simulink library "carnot"  (R2013b)
settings: Solver=ode45  StartTime=0.0  StopTime=10.0  RelTol=1e-3
undefined symbols (not defined in the file or in its folder): A, acol, Ahabit, Awin, Azimuth_Angle, AziWin, B, C, c1, c4, capc, caph, CarnotCallbacks_Density, CarnotCallbacks_Enthalpy, CarnotCallbacks_Enthalpy2Temperature, CarnotCallbacks_Entropy, CarnotCallbacks_Evaporation_Enthalpy, CarnotCallbacks_GlobalMessageLevel, CarnotCallbacks_Grashof, CarnotCallbacks_Heat_Capacity, CarnotCallbacks_Kinematic_Viscosity, CarnotCallbacks_Prandtl, CarnotCallbacks_Saturation_Property, CarnotCallbacks_Saturation_Temperature, CarnotCallbacks_Saturation_Value_Water, CarnotCallbacks_Specific_Volume, CarnotCallbacks_Thermal_Conductivity, CarnotCallbacks_Vapour_Content, CarnotCallbacks_Vapour_Pressure, con, cond, d, Dd, density, dfin, dia, DiameterLastPiece, DPConstant, dpipe, DPLinear, DPQuadratic, emission_out, fluid, FluidMix, FluidType, FPC, frame, g, GeodeticHeight, Gwin, heat_capacity, hgt, HP, Hroom, ID, inlet, K, l, lin, lpipe ... (+29)
undefined symbols (not defined in the file): c2, c3, c5, c6, cwall, dactive, height, mc, mID, rho, tau, UAneighbour, UAwall, uloss
libraries: carnot x333, simulink x25, simulink_extras x7
(part 2 of 16)

== system carnot/Source ==
  Boiler : Subsystem
      mask Display: plot(-20,0,120,100,[10,90,90,10,10],[10,10,20,20,10],[80,80,20,20],[20,90,90,20],[20,70,70,20],[24,24,30,30],[32,30,28],[30,40,30],[43,40,38],[30,40,30],[53,50,47],[30,40,30],[63,60,57],[30,40,30],[35,32,30,29,31,36,39,40,37,35],[75,69,65,58,50,49,53,59,68,75],[57,54,51,51,53,58,62,62,59,57],[76,71,67,58,49,48,54,60,69,76])
  Chiller : Subsystem
      mask Display: plot(0,0,100,100,[10,10,40,40,10],[10,40,40,10,10],[50,70,90,50],[30,65,30,30],[20,10,10,20,30,40,40,30,20],[50,60,70,80,80,70,60,50,50])
  Electric_Generator : Subsystem
      mask Display: plot(0,0,100,100,[40,20],[50,50],[40,40],[30,70],[50,50],[-0,100],[70,50],[50,50])
  Energy : Subsystem
      mask Display: plot(0,0,100,100,[10,10,40,40,10],[10,40,40,10,10],[50,70,90,50],[30,65,30,30],[20,10,10,20,30,40,40,30,20],[50,60,70,80,80,70,60,50,50])
  Heat_Exchanger : Subsystem
      mask Display: plot(0,0,100,100,[70,30,30,70,70,30],[90,10,90,90,10,10])
  Heat_Pump : Subsystem
      mask Display: plot(20,20,80,100,[30,46,36,46,36,46,30],[40,40,50,60,70,80,80],[70,54,64,54,64,54,64,54,64,54,70],[40,40,44,50,55,60,65,70,75,80,80],[56,45],[95,95],[51,51],[82,95])
  Simple : Subsystem
      mask Display: plot(0,0,100,100,[30,40,60,70,70,30,30],[50,44,44,50,10,10,50],[50,50],[44,57],[50,46,44,46,50,54,56,54,50],[93,85,70,54,48,54,70,85,93])
  Solar_Thermal : Subsystem
      mask Display: plot(0,0,100,100,[0,10,16,19,20],[80,81,84,90,100],[7,10],[79,60],[17,30],[84,70],[21,40],[94,90],[30,90,100,40,30],[10,70,60,-0,10],[90,90,40,33],[70,60,10,13],[89,39],[61,12])
  Ventilation : Subsystem
      mask Display:
      | plot([0.2 0.35], [0.8 0.7])
      | plot([0.35 0.65], [0.7 0.7])
      | plot([0.65 0.8], [0.7 0.8])
      | plot([0.65 0.8], [0.76 0.8])
      | plot([0.7 0.8], [0.65 0.8])
      | plot([0.2 0.35], [0.2 0.3])
      | plot([0.35 0.65], [0.3 0.3])
      | plot([0.65 0.8], [0.3 0.2])
      | plot([0.2 0.25], [0.2 0.32])
      | plot([0.2 0.35], [0.2 0.23])
      | plot ([0.45 0.45], [0 1])
      | plot ([0.55 0.55], [0 1])
      | plot ([0.45 0.55], [0.2 0.2])
      | plot ([0.45 0.55], [0.8 0.8])
      | plot ([0.45 0.55], [0 0.2])
      | plot ([0.45 0.55], [0.8 1])

== system carnot/Storage ==
  Thermal : Subsystem
      mask Display: plot(30,40,60,90,[36,36,40,50,54,54,50,40,36],[90,50,45,45,50,90,93,93,90],[36,51,40,51,36],[74,74,79,85,85],[36,51,44,51,36],[54,54,56,58,58])

== system carnot/Toolbox ==
  Average : Subsystem  mask{time_intervall=1 h, offset_flag=on, enable_flag=on}
      mask prompts: time_intervall "Delta t"; offset_flag "start calculating every full hour"; enable_flag "only calculate when enabled"
      mask help:
      | This block calculates the average of each input vector during a specified time Delta_t. During this time interval the output is held.
      | The output time is the time of the last average calculation.
      |  Every time the average is calculated again, a signal pulse of 1 is put out.
      |
      | When the full hour flag is set, the calculation of the average is started every full hour once again.
      |
      | When the enable flag is set, the functions calculates only while the enable signal is 1. When it is 0, the function repeats putting out the last output.
      mask init:
      | time_list = [3600 1800 900 600 300];
      | delta_t = time_list(time_intervall);
      mask Help: web(fullfile(path_carnot('help'),'Average.html'),'-helpbrowser')
      mask TypeOptions time_intervall: 1 h | 30 min | 15 min | 10 min | 5 min
  Count_Working_Time : S-Function  FunctionName=countcycles  EnableBusSupport=off  mask(count working time){}
      mask help: This block counts the number of on cycles and the working time (time when input is above zero).
      mask Help: web(fullfile(path_carnot('help'),'Count_Working_Time.html'),'-helpbrowser')
      mask Display:
      | port_label('input', 1, 'Input')
      | port_label('output', 1, 'flank')
      | port_label('output', 2, 'cycles')
      | port_label('output', 3, 'actual worktime')
      | port_label('output', 4, 'total worktime')
  Date2Sec : S-Function  FunctionName=date2sec_s  EnableBusSupport=off
      mask help:
      | This function calculates for a given date the sum of seconds in the year.
      | The input Year is a dummy argument.
      | 0 s is january, 1st at 0:00:00.
      |
      | INPUT VECTOR:
      | date [year month day hour minute second]
      |
      | OUTPUT VECTOR:
      | date [s]
  Economy_Ecology : Subsystem  mask(economy_ecology){}
      mask help: Calculates massflow, costs, exhaust gas etc.
      mask Help: web(fullfile(path_carnot('help'),'economy_ecology.html'),'-helpbrowser')
  GlobalMessageLevel : Subsystem  LoadFcn=CarnotCallbacks_GlobalMessageLevel('LoadFcn');  mask(Global Message Level){GLOBALLOCAL=local, DEBUGLEVEL=DEBUG, MAXTOTALWARNINGS=inf, MAXCONSECUTIVEWARNINGS=inf, WRITETOFILE=0, FILENAME='error.txt'}
      mask prompts: GLOBALLOCAL "message settings"; DEBUGLEVEL "message level"; MAXTOTALWARNINGS "maximum total number of warnings"; MAXCONSECUTIVEWARNINGS "maxmum consecutive warnings"; WRITETOFILE "write messages to file"
      mask help:
      | This block sets the message level of the complete model. Error messages and warnings are generated for example by the material properties functions (density, ...), see library Basic/Material_Properties for the blocks.
      | local - settings are defined by each block individually
      | global - settings are defined by this GlobalMessageLevel block
      | Copy this block once in the model if you want to use a global handling of Carnot error messages.
      mask init:
      | CarnotCallbacks_GlobalMessageLevel('SetData');
      mask TypeOptions GLOBALLOCAL: global | local
      mask Callback GLOBALLOCAL: CarnotCallbacks_GlobalMessageLevel('MaskCallback');
      mask TypeOptions DEBUGLEVEL: DEBUGLEVEL | INFOLEVEL | WARNINGLEVEL | ERRORLEVEL | FATALLEVEL | NOLEVEL
      mask Display:
      | fprintf(get_param(gcb, 'GLOBALLOCAL'));
      | fprintf(['\n\n', get_param(gcb, 'DEBUGLEVEL')]);
  RealDate : Subsystem  mask{form=year}
      mask prompts: form "Selector"
      mask help:
      | This functions puts out the system time and date:
      | Year - current year
      | Month - current month
      | Day - current day in the month (date)
      | Hour -  current hour (time)
      | Minute - current minute (of the time)
      | Second - current second (of the time)
      mask Help: web(fullfile(path_carnot('help'),'RealDate.html'),'-helpbrowser')
      mask TypeOptions form: year | month | day | hour | minute | second
  RealTime : Subsystem
      mask help:
      | This functions puts out the system time in seconds.
      | Output 0 s means January, 1st 0:00
      mask Help: web(fullfile(path_carnot('help'),'RealTime.html'),'-helpbrowser')
  RealTimePulse : Subsystem  mask{typ=rising, time=3}
      mask prompts: typ "type"; time "time interval [s]"
      mask help:
      | This functions creates a signal pulse, whenever the input pulse is
      | changing as specified. The duration of the pulse is depending on the system time, not the simulation time.
      |
      | INPUT VECTOR:
      |   in : signal to start pulse [0,1]
      |
      | OUTPUT VECTOR:
      |  out : new pulse [0,1]
      mask Help: web(fullfile(path_carnot('help'),'RealTimePulse.html'),'-helpbrowser')
      mask TypeOptions typ: rising | falling | either
  Sec2Date : S-Function  FunctionName=sec2date_s  EnableBusSupport=off
      mask help:
      | This functions calculates from a given number of seconds the date.
      |
      | INPUT VECTOR:
      | - time [s]
      |
      | OUTPUT VECTOR:
      | - date [month day hour minute second]
  SumTime : S-Function  FunctionName=sumtime_s  EnableBusSupport=off
      mask help:
      | This function calcultes for a given date the sum of seconds, minutes, ... in the year.
      |
      | INPUT VECTOR:
      | date [year month day hour minute second]
      |
      | OUTPUT VECTOR:
      | sum of |year month day hour minute second]
      mask Help: web(fullfile(path_carnot('help'),'SumTime.html'),'-helpbrowser')
      mask Display: plot(0,0,70,60,[40 20 35 20 40],[50 50 30 10 10],[50 50 45 55 50  50 52 54],[45 35 35 35 35 20 17 15]);
  SystemPulse : Subsystem  mask(system pulse){enable_flag=on, datecheck=off, date=[2 10 10 36 15], period=5, pulsewidth=2}
      mask prompts: enable_flag "Wait for enabling pulse"; datecheck "Wait for start date"; date "start date [month day hour minute second]"; period "period [s]"; pulsewidth "pulse width [s]"
      mask help:
      | This block generates a discrete pulse of 0 and 1, but this pulse depends on the system time, not the simulation time.
      | If the date flag is set, the function starts pulsing only when the system date reaches the specified date. Otherwise the output is 0.
      | If the enable flag is set, the function waits, until the enabling pulse once rise from 0 to 1. Afterwards the pulsing is started. Before pulsing the output will be 0.
      mask Help: web(fullfile(path_carnot('help'),'SystemPulse.html'),'-helpbrowser')
  THB2THV : Subsystem  InitFcn=load('THB.mat');  mask(THB2THV){}
      mask help: This block converts the Thermo-Hydraulic-Bus to the old Thermo-Hydraulic-Vector.
      mask Help: web(fullfile(path_carnot('help'),'THB2THV.html'),'-helpbrowser')
  THBMemory : Subsystem  InitFcn=load('THB.mat');  mask(THB Memory){ID=20001, T=20, mdot=0, p=1e5, FluidType=1, FluidMix=0, d=0.01, c=0, l=0, q=0, LH=1000, H=0, Annotation_ID=off, Annotation_T=off, Annotation_mdot=off, Annotation_p=off, Annotation_FluidType=off, Annotation_FluidMix=off, Annotation_d=off, Annotation_c=off, Annotation_l=off, Annotation_q=off, Annotation_LH=off, Annotation_H=off}
      mask prompts: ID "Fluid ID [1]"; T "Temperature [°C]"; mdot "Mass flow rate [kg/s]"; p "Pressure [Pa]"; FluidType "Fluid type [enum]"; FluidMix "Fluid mix [1]"; d "Diameter of the last piece [m]"; c "Constant pressure drop coefficient [Pa]"; l "Linear pressure drop coefficient [Pa/(kg/s)]"; q "Quadratic pressure drop coefficient [Pa/(kg/s)²]"; LH "Hydraulic inductance [1/m]"; H "Geodetic height [m]"; Annotation_ID "Fluid ID as annotation"; Annotation_T "Temperature as annoation"; Annotation_mdot "Mass flow rate as annoation"; Annotation_p "Pressure as annotation"; Annotation_FluidType "Fluid type as annotation"; Annotation_FluidMix "Fluid mix as annotation"; Annotation_d "Diameter of the last piece as annotation"; Annotation_c "Constant pressure drop coefficient as annotation"; Annotation_l "Linear pressure drop coefficient as annotation"; Annotation_q "Quadratic pressure drop coefficient as annotation"; Annotation_LH "Hydraulic inductance as annotation"; Annotation_H "Geodetic height as annotation"
      mask help: This is a memory block for a complete THB.
      mask init:
      | %annotations    
      | MaskValues=get_param(gcb,'MaskValues');
      | AnnotationString='';
      | if strcmp(MaskValues{13},'on') %ID
      |     if ~isempty(AnnotationString)
      |         AnnotationString=[AnnotationString,sprintf('\n')];
      |     end
      |     AnnotationString=[AnnotationString,'ID ',MaskValues{1}];
      | end
      |     
      | if strcmp(MaskValues{14},'on') %T
      |     if ~isempty(AnnotationString)
      |         AnnotationString=[AnnotationString,sprintf('\n')];
      |     end
      |     AnnotationString=[AnnotationString,MaskValues{2}, ' °C temperature'];
      | end
      |     
      | if strcmp(MaskValues{15},'on') %T
      |     if ~isempty(AnnotationString)
      |         AnnotationString=[AnnotationString,sprintf('\n')];
      |     end
      |     AnnotationString=[AnnotationString,MaskValues{3}, ' kg/s mass flow rate'];
      | end
      |     
      | if strcmp(MaskValues{16},'on') %p
      |     if ~isempty(AnnotationString)
      |         AnnotationString=[AnnotationString,sprintf('\n')];
      |     end
      |     AnnotationString=[AnnotationString,MaskValues{4}, ' Pa pressure'];
      | end
      | 
      | if strcmp(MaskValues{17},'on') %type
      |     if ~isempty(AnnotationString)
      |         AnnotationString=[AnnotationString,sprintf('\n')];
      |     end
      |     AnnotationString=[AnnotationString,'fluid type ',MaskValues{5}];
      | end
      |     
      | if strcmp(MaskValues{18},'on') %mix
      |     if ~isempty(AnnotationString)
      |         AnnotationString=[AnnotationString,sprintf('\n')];
      |     end
      |     AnnotationString=[AnnotationString,MaskValues{6}, ' fluid mix'];
      | end
      |     
      | if strcmp(MaskValues{19},'on') %d
      |     if ~isempty(AnnotationString)
      |         AnnotationString=[AnnotationString,sprintf('\n')];
      |     end
      |     AnnotationString=[AnnotationString,MaskValues{7}, ' m diameter last piece'];
      | end
      |     
      | if strcmp(MaskValues{20},'on') %c
      |     if ~isempty(AnnotationString)
      |         AnnotationString=[AnnotationString,sprintf('\n')];
      |     end
      |     AnnotationString=[AnnotationString,MaskValues{8}, ' Pa constant pressure loss coefficient'];
      | end
      |     
      | if strcmp(MaskValues{21},'on') %l
      |     if ~isempty(AnnotationString)
      |         AnnotationString=[AnnotationString,sprintf('\n')];
      |     end
      |     AnnotationString=[AnnotationString,MaskValues{9}, ' Pa/(kg/s) linear pressure loss coefficient'];
      | end
      |     
      | if strcmp(MaskValues{22},'on') %q
      |     if ~isempty(AnnotationString)
      |         AnnotationString=[AnnotationString,sprintf('\n')];
      |     end
      |     AnnotationString=[AnnotationString,MaskValues{10}, ' Pa/(kg/s)² quadratic pressure loss coefficient'];
      | end
      |     
      | if strcmp(MaskValues{23},'on') %LH
      |     if ~isempty(AnnotationString)
      |         AnnotationString=[AnnotationString,sprintf('\n')];
      |     end
      |     AnnotationString=[AnnotationString,MaskValues{11}, ' 1/m hydraulic inductance'];
      | end
      |     
      | if strcmp(MaskValues{24},'on') %H
      |     if ~isempty(AnnotationString)
      |         AnnotationString=[AnnotationString,sprintf('\n')];
      |     end
      |     AnnotationString=[AnnotationString,MaskValues{12}, ' m geodetic height'];
      | end
      |     
      | set_param(gcb,'AttributesFormatString',AnnotationString);
      | 
      | clear MaskValues AnnotationString;
      mask Help: web(fullfile(path_carnot('help'),'THBMemory.html'),'-helpbrowser')
  THV2THB : Subsystem  InitFcn=load('THB.mat');  mask(THV2THB){}
      mask help: This block converts the old Thermo-Hydraulic-Vector to the Thermo-Hydraulic-Bus.
      mask Help: web(fullfile(path_carnot('help'),'THV2THB.html'),'-helpbrowser')
  UnitConv : Subsystem  mask{input_unit='kW/(m*h)', output_unit='W/(cm*min)'}
      mask prompts: input_unit "input unit"; output_unit "output unit"
      mask help:
      | This function converts the input from a specified unit to another specified unit.
      |   When specifying a unit, the unit symbols have to be separated by * or /.
      |   That means kWh has to be written as kW*h.
      |
      | INPUT VECTOR
      |   in : value of input unit
      |
      | OUTPUT VECTOR
      |   out : input value converted to value of output unit
      mask Help: web(fullfile(path_carnot('help'),'UnitConv.html'),'-helpbrowser')
  UnitConv_Temperature : Subsystem  mask(temperature unit conversion){ini_unit=°C, fin_unit=°F}
      mask prompts: ini_unit "initial unit of the temperature"; fin_unit "target unit of the temperature"
      mask help:
      | converts a temperature form a unit to another.
      |
      | initial unit and target unit should be one of the following characters :
      |   - '°C' : Celsius
      |   - 'K' : Kelvin
      |   - '°F' : Farenheit
      |
      | Warning : a difference of temperature doesn't need to be convert from
      | Kelvin to Celsius.
      mask Help: web(fullfile(path_carnot('help'),'UnitConv_Temperature.html'),'-helpbrowser')
      mask TypeOptions ini_unit: °C | K | °F
      mask TypeOptions fin_unit: °C | K | °F
  WDB2Weather : Subsystem  mask(WDB 2 weather){}
      mask help:
      | Creates the weather data vector from the weather data bus WDB.
      | Format in weather data vector:
      | 1  timevalue (comment line) format YYYYMMDDHHMM    -
      | 2  zenith angle of sun (at time, not averaged)       degree
      | 3  azimuth angle of sun (0°=south, east negative) degree
      | 4  beam solar radiation on a normal surface         W/m^2
      | 5  diffuse solar radiation on a horizontal surface   W/m^2
      | 6  ambient temperature                                    degree celsius
      | 7  radiation temperature of sky                          degree celsius
      | 8  relative humidity                                           percent
      | 9  precipitation                                                 m/s
      | 10 cloud index (0=no cloud, 1=covered sky)         -
      | 11 station pressure                                           Pa
      | 12 mean wind speed                                         m/s
      | 13 wind direction (north=0° west=270°)             degree
      | 14 incidence angle on surface (0° = vertical)      degree
      | 15 longitudinal incidence angle                       degree
      | 16 transversal incidence angle                        degree
      | 17 direct solar radiation on surface                 W/m²
      | 18 diffuse solar radiation on surface                W/m²
  Wait : Subsystem  mask{check=off, date=[1 10 15 31 00], wtime=1}
      mask prompts: check "Look for start date"; date "start date [month day hour minute second]"; wtime "waiting time [s]"
      mask help:
      | This function waits until the system time reaches the given date.
      | Whenever called again, this function will wait for the given number of seconds.
      mask init:
      | if check==0
      |  date(1) = -1;
      | end;
      mask Help: web(fullfile(path_carnot('help'),'Wait.html'),'-helpbrowser')
      mask Display: plot(-31,-31,31,31,[0     9    17    23    28    30    29    26    20    13     4    -5 -13   -21   -26   -29   -30   -28   -23   -17    -8 1],[ 30    29    25    19    11     2    -7   -15   -22   -27   -30   -30 -27   -22   -15    -6     3    11    19    25    29 30],[-20,0,0],[0,0,20])
  Weather2WDB : Subsystem  mask(weather 2 WDB){}
      mask help:
      | Creates the weather data bus WDB from the weather data vector.
      | Format in weather data vector:
      | 1  timevalue (comment line) format YYYYMMDDHHMM    -
      | 2  zenith angle of sun (at time, not averaged)       degree
      | 3  azimuth angle of sun (0°=south, east negative) degree
      | 4  beam solar radiation on a normal surface         W/m^2
      | 5  diffuse solar radiation on a horizontal surface   W/m^2
      | 6  ambient temperature                                    degree celsius
      | 7  radiation temperature of sky                          degree celsius
      | 8  relative humidity                                           percent
      | 9  precipitation                                                 m/s
      | 10 cloud index (0=no cloud, 1=covered sky)         -
      | 11 station pressure                                           Pa
      | 12 mean wind speed                                         m/s
      | 13 wind direction (north=0° west=270°)             degree
      | 14 incidence angle on surface (0° = vertical)      degree
      | 15 longitudinal incidence angle                       degree
      | 16 transversal incidence angle                        degree
      | 17 direct solar radiation on surface                 W/m²
      | 18 diffuse solar radiation on surface                W/m²
  write_txt_file : Subsystem  mask{clear=off, filename='testout.txt'}
      mask prompts: clear "clear existing file"
      mask help:
      | This function writes the input data to a ascii-txt-file, so it can be opened with an usual editor.
      | The data is only written, when the enable signal is 1.
      | It's possible to append data to an existing file or to clear the file before writing.
      |
      | INPUT VECTOR
      |   in         : input data
      |   enable : signal [0,1]
      mask Help: web(fullfile(path_carnot('help'),'write_txt_file.html'),'-helpbrowser')

== system carnot/Weather ==
  Add_Solar_Position : Subsystem  mask(sun position){longi=-7, lati=50, timezone=-15}
      mask prompts: longi "geographical longitude [degrees] (east negative)"; lati "geographical latitude [degrees] (north positive)"; timezone "longitude of timezone [degrees] (east negative)"
      mask help:
      | This funktion calculates the sun position  and sets it in the weather data vector. Solar zenith angle and azimuth angle (in degrees) (east negative, south = 0°) are set in the weather vector.
      | Timezones:    GMT = 0
      |                       MEZ = -15
      |                       MESZ = -30
      mask init:
      | longi = min(180, max(-180, longi));
      | lati = min(90, max(-90, lati));
      | timezone = min(360, max(-360, timezone));
      mask Help: web(fullfile(path_carnot('help'),'Solar_Position.html'),'-helpbrowser')
  DWD_TRY_Radiation_Filter : Subsystem  mask(DWD TRY Filter){f=5}
      mask prompts: f "Filter llevel (1 = high, 10 = low)"
      mask help:
      | Filter for solar beam radiation of test reference years 2010 of the german DWD.
      | The original data has some defaults which results in a wrong time-vector (and solar position).
      mask Help: web(fullfile(path_carnot('help'),'DWD_TRY_Radiation_Filter.html'),'-helpbrowser')
  Fixed_Surface : Subsystem  mask(fixed surface){colangle=30, colazi=0, colrot=0}
      mask prompts: colangle "collector slope (0° = horizontal) [degree]"; colazi "collector azimuth (0° = south, -90° = east) [degree]"; colrot "collector rotation angle [degree]"
      mask help:
      | Set collector or surface to a fixed position.
      | All angles in degrees.
      mask init:
      | colangle = min(180, max(-180, colangle));
      | colazi = min(180, max(-180, colazi));
      | colrot = min(180, max(-180, colrot));
      mask Help: web(fullfile(path_carnot('help'),'Fixed_Surface.html'),'-helpbrowser')
  Radiation_on_Inclined_Surface : Subsystem  mask(inclined surface){sky=Perez 1990, reflect=0.2}
      mask prompts: sky "sky model"; reflect "ground reflectance (0..1)"
      mask help: Calculates the radiation on inclined surfaces from sun-position (zenith angle and azimuth). The radiation and incidence angles for the inclined surface are set in the weather vector. All angles are in degrees.
      mask init:
      | reflect = min(1.0, max(0.0, reflect));
      mask Help: web(fullfile(path_carnot('help'),'Radiation_on_Inclined_Surface.html'),'-helpbrowser')
      mask TypeOptions sky: isotropic sky | Hay-Davies | Perez 1990
  Select_Weather : Subsystem  mask(Select weather data){v=[6 7]}
      mask prompts: v "vector of index"
      mask help:
      | Selects the indexed weather data from the input weather data vector.
      | Format in weather data vector:
      | 1  timevalue (comment line) format YYYYMMDDHHMM    -
      | 2  zenith angle of sun (at time, not averaged)       degree
      | 3  azimuth angle of sun (0°=south, east negative) degree
      | 4  beam solar radiation on a normal surface         W/m^2
      | 5  diffuse solar radiation on a horizontal surface   W/m^2
      | 6  ambient temperature                                    degree celsius
      | 7  radiation temperature of sky                          degree celsius
      | 8  relative humidity                                           percent
      | 9  precipitation                                                 m/s
      | 10 cloud index (0=no cloud, 1=covered sky)         -
      | 11 station pressure                                           Pa
      | 12 mean wind speed                                         m/s
      | 13 wind direction (north=0° west=270°)             degree
      | 14 incidence angle on surface (0° = vertical)      degree
      | 15 longitudinal incidence angle                       degree
      | 16 transversal incidence angle                        degree
      | 17 direct solar radiation on surface                 W/m²
      | 18 diffuse solar radiation on surface                W/m²
      mask Help: eval('man(''select_weather'')')
  Tracked_Surface : Subsystem  mask(tracked surface){tracktype=two axis tracking, inc=0, azi=0, rot=0, time=0}
      mask prompts: tracktype "tracking type"; inc "inclination of surface or axis [degrees]"; azi "azimuth of surface or axis (0° = south, -90° = east) [degree]"; rot "rotation of surface or axis [degree]"; time "tracking time [s]"
      mask help: Performs a collector tracking around a given axis. You may specify the time in seconds between two trackings.
      mask Help: web(fullfile(path_carnot('help'),'Tracked_Surface.html'),'-helpbrowser')
      mask TypeOptions tracktype: axis is collector riser | vertical axis | two axis tracking | fixed surface
  WDB2THB : Subsystem  mask(Weather Data Bus to Thermo Hydraulic Bus){dia=0.2}
      mask prompts: dia "diameter [m]"
      mask help: Transfers the incoming weather data to an air flow in the thermo-hydraulic vector THV. All properties are set to ambient conditions (temperature, pressure, humidity).
      mask init:
      | dia = max(dia, 0.001);
      mask Help: web(fullfile(path_carnot('help'),'WDB2THB.html'),'-helpbrowser')
  Weather_Simple_Model : Subsystem  mask(Weather Simple Model){lat=60, Ibn=900, Idg=100, tamb=5, deltaTsky=-6, rh=50, precip=10e-3/24/3600           % 10 mm in 24 h, cloud=0.125, p=1013e2, vw=1, wdir=270}
      mask prompts: lat "Latitude in degree (north positve)"; Ibn "Maximum beam radiation on normal surface in W/m²"; Idg "Maximum diffuse radiation on horizontal surface in W/m²"; tamb "Ambient temperature in °C"; deltaTsky "Offset for sky temperature in K (usually -6K)"; rh "Relative humidity in %"; precip "Rainfall (precipitation) in m/s"; cloud "Cloud index in (0..1)"; p "Air pressure in Pa"; vw "Wind speed in m/s"; wdir "Wind direction in ° (0° = North, 90° = East)"
      mask help:
      | Create a simple, mostly constant weather data bus (WDB).
      | The solar radiation corresponds to clear sky conditions.
      mask Help: web(fullfile(path_carnot('help'),'Weather_Simple_Model.html'),'-helpbrowser')
  Weather_from_File : Subsystem  mask(weather from file){file=DE_TRY2010_04_averageYear, ext=.mat}
      mask prompts: file "Name of file"; ext "Extension of file"
      mask help:
      | Input block for external weather data files. The file is read to the workspace. A "From Workspace" Block is used in the subsystem.
      | A Unit-Delay with the timestep of the weather data forces the model to a maximum timestep equal to the data acquisiton timestep.
      | Remark: Be carefull when using the TRY Data 2010 for Germany. The files are public and can be found in the parameter_set folder of this block. But there are bugs is the solar radiation data.
      mask init:
      | % path definitions
      | parampath = fullfile('Weather','Weather_from_File','parameter_set');
      | 
      | CarnotCallbacks_GetFiles;
      | 
      | % filename = [file, ext];
      | % intfile = fullfile(path_carnot('intlibsl'), parampath, filename);
      | % pubfile = fullfile(path_carnot('libsl'), parampath, filename);
      | % 
      | % if ~BlockIsInCarnotLibrary          % not in carnot library any more
      | %     if exist(filename,'file')       % search file on matlab path
      | %         evalin('base',['load(''' filename ''');'])
      | %     elseif exist(intfile,'file')    % search on internal path
      | %         evalin('base',['load(''' intfile ''');'])
      | %     elseif exist(pubfile,'file')    % search on public path
      | %         evalin('base',['load(''' pubfile ''');'])
      | %     end
      | %     set_param([gcb '/From_Workspace'], 'VariableName', file);
      | % end
      | % 
      | % % sample time is timestep of weather data
      | % rawdata = load(file);
      | % varnames = fieldnames(rawdata);
      | % t_sample = rawdata.(varnames{1})(3,1) - rawdata.(varnames{1})(2,1);
      | % clear rawdata;
      | % clear varnames;
      mask Help: web(fullfile(path_carnot('help'),'weather_from_file.html'),'-helpbrowser')
      mask TypeOptions ext: .dat | .txt | .mat
      mask Display: disp(file)
  Weather_from_Workspace : Subsystem  mask(weather from workspace){file=DE_TRY2010_06_averageYear}
      mask prompts: file "Name of variable"
      mask help:
      | Input block for external weather data variables. The variable must be available in the workspace. A "From Workspace" Block is used in the subsystem.
      | A Unit-Delay with the timestep of the weather data forces the model to a maximum timestep equal to the data acquisiton timestep.
      | Remark: Be carefull when using the TRY Data 2010 for Germany. The files are public and can be found in the parameter_set folder of this block. But there are bugs is the solar radiation data.
      mask init:
      | % set variable name in the From Workspace block
      | set_param([gcb '/From_Workspace'], 'VariableName', file);
      | 
      | 
      | t_sample = evalin('base',eval(['''',eval('file'),'(3,1)'''])) - evalin('base',eval(['''',eval('file'),'(2,1)''']));
      | % sample time is timestep of weather data
      | %evalin('caller',['t_sample = ' file '(3,1) - ' file '(2,1);']);
      mask Help: web(fullfile(path_carnot('help'),'Weather_from_Workspace.html'),'-helpbrowser')
      mask Display: disp(file)

== system carnot/examples ==
